simulink model "LAB05_B"  (R2023b)
settings: Solver=VariableStepAuto  StartTime=0.0  StopTime=1  RelTol=1e-3
libraries: spsRMSLib x3, spsACVoltageSourceLib x1, spsCurrentMeasurementLib x1, spsLinearTransformerLib x1, spsPowerLib x1, spsVoltageMeasurementLib x1, sps_lib x1
settings Model: Creator=sagar  LastModifiedBy=sagar

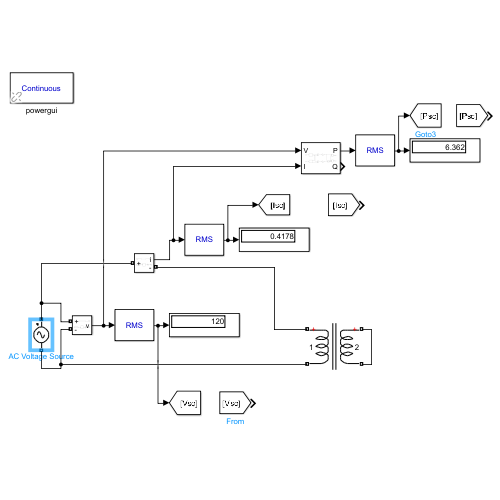
[thumbnail: Simulink's stored preview of the top-level diagram]
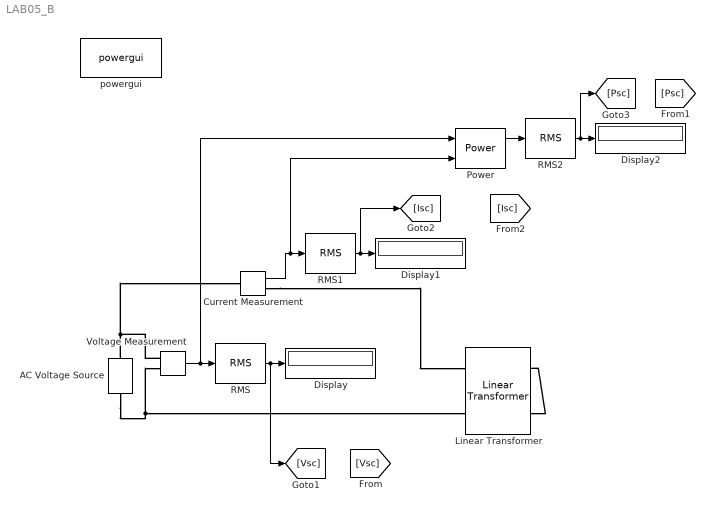
== system LAB05_B ==
  AC Voltage Source : spsACVoltageSourceLib/AC Voltage Source  Amplitude=120*sqrt(2)  Phase=0  Frequency=50  SampleTime=0.001  Measurements=None  BusType=swing  Pref=10e3  Qref=0  Qmin=-inf  Qmax=+inf
  Current Measurement : spsCurrentMeasurementLib/Current Measurement  PhasorSimulation=off  OutputType=Complex  PSBequivalent=0
  Display : Display
  Display1 : Display
  Display2 : Display
  Linear Transformer : spsLinearTransformerLib/Linear Transformer  UNITS=SI  NominalPower=[ 250e6 60 ]  winding1=[7.35e+05 4.3218 0.45856]  winding2=[3.15e+05 0.7938 0.084225]  ThreeWindings=off  winding3=[3.15e+05 0.7938 0.084225]  RmLm=[1.0804e+06 2866]  Measurements=None  DataType=on
  Power : spsPowerLib/Power  Freq=50  Vinit=[1, 0]  Iinit=[1, 0]  Ts=0.001
  RMS : spsRMSLib/RMS  TrueRMS=on  Freq=50  RMSInit=0  Ts=0.001
  RMS1 : spsRMSLib/RMS  TrueRMS=on  Freq=50  RMSInit=0  Ts=0.001
  RMS2 : spsRMSLib/RMS  TrueRMS=on  Freq=50  RMSInit=0  Ts=0.001
  Voltage Measurement : spsVoltageMeasurementLib/Voltage Measurement  PhasorSimulation=off  OutputType=Complex  PSBequivalent=0
  powergui : sps_lib/powergui  Priority=1  SimulationMode=Continuous  SampleTime=50e-6  frequency=60  Iterations=50  frequencyindice=50  Pbase=100e6  ErrMax=1e-4  UnitsV=kV  UnitsW=MW  buscounter=0  FunctionMessages=off  echomessages=off  EnableUseOfTLC=off  CurrentSourceSwitches=off  DisableSnubberDevices=off  DisableRonSwitches=off  DisableVfSwitches=off  DisplayEquations=off  AutomaticDiscreteSolvers=off  SolverType=Tustin/Backward Euler (TBE)  Interpol=off  ExternalGateDelay=off  methode=off  Ts=100  x0status=blocks  SPID=on  SwTol=0  HookPort=off  NonlinearTolerance=1e-4  nMaxIteration=100  ContinueOnMaxIteration=off  RestoreLinks=warning  ResistiveCurrentMeasurement=off  Frange=[0:2:500]  Ylog=off  Xlog=on  ShowGrid=off  save=off  variable=ZData  structure=0  ZoomFFT=off  StartTime=0.0  cycles=1  DisplayStyle=1  fundamental=60  FreqAxis=off  MaxFrequency=1000  frequencyindicesteady=1  RmsSteady=1  display=off
  wires:
  RMS/1 -> [Vsc], Display/1
  Voltage Measurement/1 -> Power/1, RMS/1
  RMS1/1 -> [Isc], Display1/1
  Current Measurement/1 -> Power/2, RMS1/1
  RMS2/1 -> [Psc], Display2/1
  Power/1 -> RMS2/1
  connections:
  AC Voltage Source/RConn1 -- Current Measurement/LConn1 -- Voltage Measurement/LConn1
  AC Voltage Source/LConn1 -- Voltage Measurement/LConn2 -- Linear Transformer/LConn2
  Current Measurement/RConn1 -- Linear Transformer/LConn1
  Linear Transformer/RConn2 -- Linear Transformer/RConn1
